simulink model "VehV"  (R2016b)
settings: Solver=VariableStepAuto  StartTime=0.0  StopTime=10.0  RelTol=1e-3
settings Model: Creator=jiakui  LastModifiedBy=jiakui

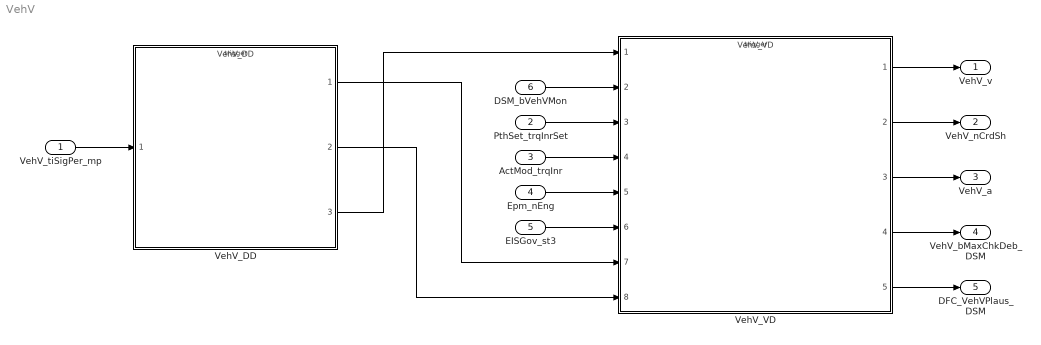
== system VehV ==
  VehV_tiSigPer_mp : Inport  Tag=us  Description=signal period duration  OutMin=0  OutMax=6553  OutDataTypeStr=Period_us
  PthSet_trqInrSet : Inport  Tag=Nm  Description=Inner torque set value after monitoring limitation  Port=2  OutMin=-3000  OutMax=3276.7  OutDataTypeStr=Trq_Nm
  ActMod_trqInr : Inport  Tag=Nm  Description=Current, back-calculated inner engine torque  Port=3  OutMin=-3276.8  OutMax=3276.7  OutDataTypeStr=Trq_Nm
  Epm_nEng : Inport  Tag=rpm  Description=Engine speed  Port=4  OutMin=0  OutMax=6000  OutDataTypeStr=EngSpeed_rpm
  EISGov_st3 : Inport  Description=Status information of WESDem client  Port=5  OutMin=0  OutMax=2147483648  OutDataTypeStr=State_uint32
  DSM_bVehVMon : Inport  Description=state of FId_VehVMon  Port=6  OutMin=0  OutMax=1  OutDataTypeStr=boolean
  VehV_DD : ModelReference  ModelNameDialog=VehV_DD  SimulationMode=Normal  ModelReferenceVersion=1.5  TriggerPortName=function  TriggerPortTriggerType=function-call  TriggerPortStatesWhenEnabling=held
  VehV_VD : ModelReference  ModelNameDialog=VehV_VD  SimulationMode=Normal  ModelReferenceVersion=1.8  TriggerPortName=function  TriggerPortTriggerType=function-call  TriggerPortStatesWhenEnabling=held
  VehV_v : Outport  Tag=km/h  Description=Vehicle speed  OutMin=0  OutMax=250  OutDataTypeStr=VehSpeed_km_h
  VehV_nCrdSh : Outport  Tag=rpm  Description=Cardan shaft speed  Port=2  OutMin=0  OutMax=6000  OutDataTypeStr=EngSpeed_rpm
  VehV_a : Outport  Tag=m/s^2  Description=The acceleration of the vehicle  Port=3  OutMin=-32.7  OutMax=32.7  OutDataTypeStr=Acc_m_s2
  VehV_bMaxChkDeb_DSM : Outport  Description=status of VehV_bMaxChkDeb  Port=4  OutMin=0  OutMax=1  OutDataTypeStr=boolean
  DFC_VehVPlaus_DSM : Outport  Description=state of DFC_VehVPlaus  Port=5  OutMin=0  OutMax=1  OutDataTypeStr=boolean
  wires:
  VehV_tiSigPer_mp/1 -> VehV_DD/1
  VehV_DD/3 -> VehV_VD/1
  VehV_DD/1 -> VehV_VD/7
  VehV_DD/2 -> VehV_VD/8
  PthSet_trqInrSet/1 -> VehV_VD/3
  ActMod_trqInr/1 -> VehV_VD/4
  Epm_nEng/1 -> VehV_VD/5
  EISGov_st3/1 -> VehV_VD/6
  VehV_VD/1 -> VehV_v/1
  VehV_VD/2 -> VehV_nCrdSh/1
  VehV_VD/3 -> VehV_a/1
  VehV_VD/5 -> DFC_VehVPlaus_DSM/1
  VehV_VD/4 -> VehV_bMaxChkDeb_DSM/1
  DSM_bVehVMon/1 -> VehV_VD/2
